simulink model "timer_load_8bit"  (R2016a)
settings: Solver=VariableStepAuto  StartTime=0.0  StopTime=1028  RelTol=1e-3
libraries: simulink_extras x9
settings Model: Creator=Cosmin  LastModifiedBy=Cosmin

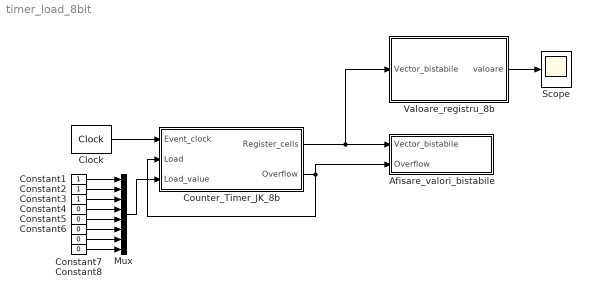
== system timer_load_8bit ==
  Afisare_valori_bistabile : Subsystem
  Clock : simulink_extras/Flip Flops/Clock  period=2
  Constant1 : Constant  OutDataTypeStr=boolean
  Constant2 : Constant  OutDataTypeStr=boolean
  Constant3 : Constant  OutDataTypeStr=boolean
  Constant{4..8} (5 alike) : Constant  Value=0  OutDataTypeStr=boolean
  Counter_Timer_JK_8b : Subsystem
  Mux : Mux  Inputs=8
  Scope : Scope
  Valoare_registru_8b : Subsystem
  wires:
  Valoare_registru_8b/1(valoare) -> Scope/1
  Counter_Timer_JK_8b/1(Register_cells) -> Afisare_valori_bistabile/1(Vector_bistabile), Valoare_registru_8b/1(Vector_bistabile)
  Clock/1 -> Counter_Timer_JK_8b/1(Event_clock)
  Counter_Timer_JK_8b/2(Overflow) -> Counter_Timer_JK_8b/2(Load), Afisare_valori_bistabile/2("Overflow ")
  Constant1/1 -> Mux/1
  Constant2/1 -> Mux/2
  Constant4/1 -> Mux/4
  Constant3/1 -> Mux/3
  Constant6/1 -> Mux/6
  Constant8/1 -> Mux/8
  Constant7/1 -> Mux/7
  Constant5/1 -> Mux/5
  Mux/1 -> Counter_Timer_JK_8b/3(Load_value)

== system timer_load_8bit/Afisare_valori_bistabile ==
  Vector_bistabile : Inport
  "Overflow " : Inport  Port=2
  Demux1 : Demux  Outputs=8
  Evolutie_bistabile_registru : Scope  NumInputPorts=9
  wires:
  Vector_bistabile/1 -> Demux1/1
  Demux1/4 -> Evolutie_bistabile_registru/4
  Demux1/2 -> Evolutie_bistabile_registru/2
  Demux1/1 -> Evolutie_bistabile_registru/1
  Demux1/3 -> Evolutie_bistabile_registru/3
  Demux1/7 -> Evolutie_bistabile_registru/7
  Demux1/5 -> Evolutie_bistabile_registru/5
  Demux1/6 -> Evolutie_bistabile_registru/6
  Demux1/8 -> Evolutie_bistabile_registru/8
  "Overflow "/1 -> Evolutie_bistabile_registru/9

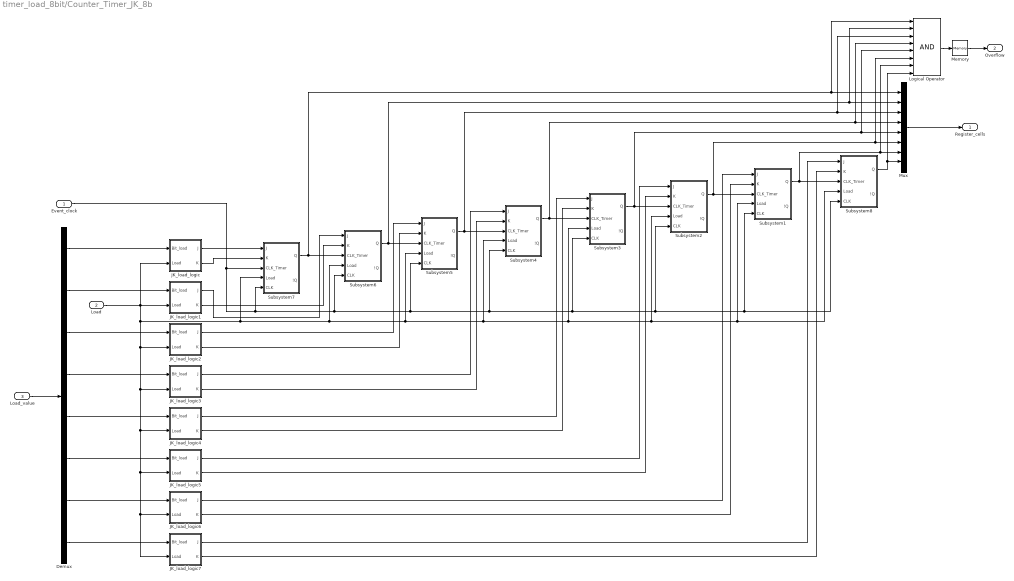
== system timer_load_8bit/Counter_Timer_JK_8b ==
  Event_clock : Inport
  Load : Inport  Port=2
  Load_value : Inport  Port=3
  Demux : Demux  Outputs=8
  JK_load_logic : Subsystem
  JK_load_logic1 : Subsystem
  JK_load_logic2 : Subsystem
  JK_load_logic3 : Subsystem
  JK_load_logic4 : Subsystem
  JK_load_logic5 : Subsystem
  JK_load_logic6 : Subsystem
  JK_load_logic7 : Subsystem
  Logical Operator : Logic  Inputs=8  AllPortsSameDT=off  OutDataTypeStr=boolean
  Memory : Memory
  Mux : Mux  Inputs=8
  Subsystem1 : Subsystem
  Subsystem2 : Subsystem
  Subsystem3 : Subsystem
  Subsystem4 : Subsystem
  Subsystem5 : Subsystem
  Subsystem6 : Subsystem
  Subsystem7 : Subsystem
  Subsystem8 : Subsystem
  Register_cells : Outport
  Overflow : Outport  Port=2
  wires:
  Mux/1 -> Register_cells/1
  Load/1 -> Subsystem7/4(Load), Subsystem6/4(Load), Subsystem5/4(Load), Subsystem4/4(Load), Subsystem3/4(Load), Subsystem2/4(Load), Subsystem8/4(Load), Subsystem1/4(Load), JK_load_logic2/2(Load), JK_load_logic3/2(Load), JK_load_logic4/2(Load), JK_load_logic5/2(Load), JK_load_logic7/2(Load), JK_load_logic6/2(Load), JK_load_logic/2(Load), JK_load_logic1/2(Load)
  Event_clock/1 -> Subsystem7/3(CLK_Timer), Subsystem7/5(CLK), Subsystem6/5(CLK), Subsystem5/5(CLK), Subsystem4/5(CLK), Subsystem3/5(CLK), Subsystem2/5(CLK), Subsystem8/5(CLK), Subsystem1/5(CLK)
  Load_value/1 -> Demux/1
  Demux/1 -> JK_load_logic/1(Bit_load)
  Demux/2 -> JK_load_logic1/1(Bit_load)
  Demux/3 -> JK_load_logic2/1(Bit_load)
  Demux/4 -> JK_load_logic3/1(Bit_load)
  Demux/5 -> JK_load_logic4/1(Bit_load)
  Demux/6 -> JK_load_logic5/1(Bit_load)
  Demux/7 -> JK_load_logic6/1(Bit_load)
  Demux/8 -> JK_load_logic7/1(Bit_load)
  JK_load_logic6/1(J) -> Subsystem1/1(J)
  JK_load_logic7/2(K) -> Subsystem8/2(K)
  JK_load_logic7/1(J) -> Subsystem8/1(J)
  Logical Operator/1 -> Memory/1
  Subsystem8/1(Q) -> Logical Operator/8, Mux/8
  Subsystem1/1(Q) -> Subsystem8/3(CLK_Timer), Logical Operator/7, Mux/7
  Subsystem2/1(Q) -> Logical Operator/6, Mux/6, Subsystem1/3(CLK_Timer)
  JK_load_logic6/2(K) -> Subsystem1/2(K)
  JK_load_logic5/1(J) -> Subsystem2/1(J)
  JK_load_logic5/2(K) -> Subsystem2/2(K)
  Subsystem3/1(Q) -> Subsystem2/3(CLK_Timer), Mux/5, Logical Operator/5
  JK_load_logic4/1(J) -> Subsystem3/1(J)
  JK_load_logic4/2(K) -> Subsystem3/2(K)
  Subsystem4/1(Q) -> Subsystem3/3(CLK_Timer), Mux/4, Logical Operator/4
  JK_load_logic3/1(J) -> Subsystem4/1(J)
  JK_load_logic3/2(K) -> Subsystem4/2(K)
  Subsystem5/1(Q) -> Subsystem4/3(CLK_Timer), Mux/3, Logical Operator/3
  JK_load_logic2/1(J) -> Subsystem5/1(J)
  JK_load_logic2/2(K) -> Subsystem5/2(K)
  Subsystem6/1(Q) -> Subsystem5/3(CLK_Timer), Logical Operator/2, Mux/2
  Subsystem7/1(Q) -> Subsystem6/3(CLK_Timer), Mux/1, Logical Operator/1
  JK_load_logic1/1(J) -> Subsystem6/1(J)
  JK_load_logic1/2(K) -> Subsystem6/2(K)
  JK_load_logic/1(J) -> Subsystem7/1(J)
  JK_load_logic/2(K) -> Subsystem7/2(K)
  Memory/1 -> Overflow/1

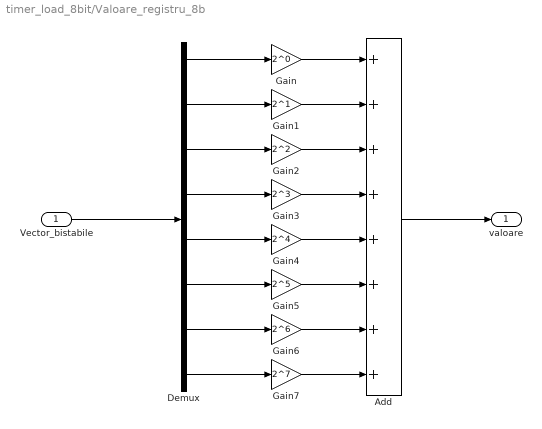
== system timer_load_8bit/Valoare_registru_8b ==
  Vector_bistabile : Inport
  Add : Sum  Inputs=++++++++
  Demux : Demux  Outputs=8
  Gain : Gain  Gain=2^0  OutDataTypeStr=uint8
  Gain1 : Gain  Gain=2^1  OutDataTypeStr=uint8
  Gain2 : Gain  Gain=2^2  OutDataTypeStr=uint8
  Gain3 : Gain  Gain=2^3  OutDataTypeStr=uint8
  Gain4 : Gain  Gain=2^4  OutDataTypeStr=uint8
  Gain5 : Gain  Gain=2^5  OutDataTypeStr=uint8
  Gain6 : Gain  Gain=2^6  OutDataTypeStr=uint8
  Gain7 : Gain  Gain=2^7  OutDataTypeStr=uint8
  valoare : Outport
  wires:
  Demux/1 -> Gain/1
  Demux/6 -> Gain5/1
  Demux/7 -> Gain6/1
  Demux/2 -> Gain1/1
  Demux/5 -> Gain4/1
  Gain5/1 -> Add/6
  Gain6/1 -> Add/7
  Gain2/1 -> Add/3
  Gain4/1 -> Add/5
  Gain3/1 -> Add/4
  Gain7/1 -> Add/8
  Gain1/1 -> Add/2
  Gain/1 -> Add/1
  Vector_bistabile/1 -> Demux/1
  Demux/3 -> Gain2/1
  Demux/4 -> Gain3/1
  Demux/8 -> Gain7/1
  Add/1 -> valoare/1

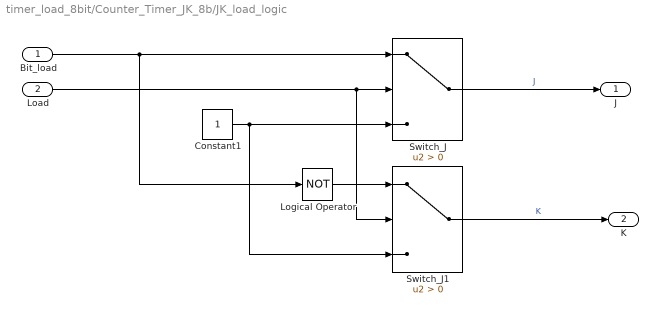
== system timer_load_8bit/Counter_Timer_JK_8b/JK_load_logic ==
  Bit_load : Inport
  Load : Inport  Port=2
  Constant1 : Constant  OutDataTypeStr=boolean
  Logical Operator : Logic  Operator=NOT  AllPortsSameDT=off  OutDataTypeStr=boolean
  Switch_J : Switch  Criteria=u2 > Threshold  OutDataTypeStr=Inherit: Inherit via back propagation
  Switch_J1 : Switch  Criteria=u2 > Threshold  OutDataTypeStr=Inherit: Inherit via back propagation
  J : Outport  OutDataTypeStr=boolean
  K : Outport  Port=2  OutDataTypeStr=boolean
  wires:
  Switch_J/1 -> J/1  "J"
  Bit_load/1 -> Logical Operator/1, Switch_J/1
  Logical Operator/1 -> Switch_J1/1
  Load/1 -> Switch_J1/2, Switch_J/2
  Constant1/1 -> Switch_J1/3, Switch_J/3
  Switch_J1/1 -> K/1  "K"

== system timer_load_8bit/Counter_Timer_JK_8b/JK_load_logic1 ==
  Bit_load : Inport
  Load : Inport  Port=2
  Constant1 : Constant  OutDataTypeStr=boolean
  Logical Operator : Logic  Operator=NOT  AllPortsSameDT=off  OutDataTypeStr=boolean
  Switch_J : Switch  Criteria=u2 > Threshold
  Switch_J1 : Switch  Criteria=u2 > Threshold
  J : Outport
  K : Outport  Port=2
  wires:
  Switch_J1/1 -> K/1  "K"
  Constant1/1 -> Switch_J/3, Switch_J1/3
  Load/1 -> Switch_J/2, Switch_J1/2
  Logical Operator/1 -> Switch_J1/1
  Bit_load/1 -> Switch_J/1, Logical Operator/1
  Switch_J/1 -> J/1  "J"

== system timer_load_8bit/Counter_Timer_JK_8b/JK_load_logic2 ==
  Bit_load : Inport
  Load : Inport  Port=2
  Constant1 : Constant  OutDataTypeStr=boolean
  Logical Operator : Logic  Operator=NOT  AllPortsSameDT=off  OutDataTypeStr=boolean
  Switch_J : Switch  Criteria=u2 > Threshold
  Switch_J1 : Switch  Criteria=u2 > Threshold
  J : Outport
  K : Outport  Port=2
  wires:
  Switch_J/1 -> J/1  "J"
  Bit_load/1 -> Logical Operator/1, Switch_J/1
  Logical Operator/1 -> Switch_J1/1
  Load/1 -> Switch_J1/2, Switch_J/2
  Constant1/1 -> Switch_J1/3, Switch_J/3
  Switch_J1/1 -> K/1  "K"

== system timer_load_8bit/Counter_Timer_JK_8b/JK_load_logic3 ==
  Bit_load : Inport
  Load : Inport  Port=2
  Constant1 : Constant  OutDataTypeStr=boolean
  Logical Operator : Logic  Operator=NOT  AllPortsSameDT=off  OutDataTypeStr=boolean
  Switch_J : Switch  Criteria=u2 > Threshold
  Switch_J1 : Switch  Criteria=u2 > Threshold
  J : Outport
  K : Outport  Port=2
  wires:
  Switch_J1/1 -> K/1  "K"
  Constant1/1 -> Switch_J/3, Switch_J1/3
  Load/1 -> Switch_J/2, Switch_J1/2
  Logical Operator/1 -> Switch_J1/1
  Bit_load/1 -> Switch_J/1, Logical Operator/1
  Switch_J/1 -> J/1  "J"

== system timer_load_8bit/Counter_Timer_JK_8b/JK_load_logic4 ==
  Bit_load : Inport
  Load : Inport  Port=2
  Constant1 : Constant  OutDataTypeStr=boolean
  Logical Operator : Logic  Operator=NOT  AllPortsSameDT=off  OutDataTypeStr=boolean
  Switch_J : Switch  Criteria=u2 > Threshold
  Switch_J1 : Switch  Criteria=u2 > Threshold
  J : Outport
  K : Outport  Port=2
  wires:
  Switch_J1/1 -> K/1  "K"
  Constant1/1 -> Switch_J/3, Switch_J1/3
  Load/1 -> Switch_J/2, Switch_J1/2
  Logical Operator/1 -> Switch_J1/1
  Bit_load/1 -> Switch_J/1, Logical Operator/1
  Switch_J/1 -> J/1  "J"

== system timer_load_8bit/Counter_Timer_JK_8b/JK_load_logic5 ==
  Bit_load : Inport
  Load : Inport  Port=2
  Constant1 : Constant  OutDataTypeStr=boolean
  Logical Operator : Logic  Operator=NOT  AllPortsSameDT=off  OutDataTypeStr=boolean
  Switch_J : Switch  Criteria=u2 > Threshold
  Switch_J1 : Switch  Criteria=u2 > Threshold
  J : Outport
  K : Outport  Port=2
  wires:
  Switch_J/1 -> J/1  "J"
  Bit_load/1 -> Logical Operator/1, Switch_J/1
  Logical Operator/1 -> Switch_J1/1
  Load/1 -> Switch_J1/2, Switch_J/2
  Constant1/1 -> Switch_J1/3, Switch_J/3
  Switch_J1/1 -> K/1  "K"

== system timer_load_8bit/Counter_Timer_JK_8b/JK_load_logic6 ==
  Bit_load : Inport
  Load : Inport  Port=2
  Constant1 : Constant  OutDataTypeStr=boolean
  Logical Operator : Logic  Operator=NOT  AllPortsSameDT=off  OutDataTypeStr=boolean
  Switch_J : Switch  Criteria=u2 > Threshold
  Switch_J1 : Switch  Criteria=u2 > Threshold
  J : Outport
  K : Outport  Port=2
  wires:
  Switch_J1/1 -> K/1  "K"
  Constant1/1 -> Switch_J/3, Switch_J1/3
  Load/1 -> Switch_J/2, Switch_J1/2
  Logical Operator/1 -> Switch_J1/1
  Bit_load/1 -> Switch_J/1, Logical Operator/1
  Switch_J/1 -> J/1  "J"

== system timer_load_8bit/Counter_Timer_JK_8b/JK_load_logic7 ==
  Bit_load : Inport
  Load : Inport  Port=2
  Constant1 : Constant  OutDataTypeStr=boolean
  Logical Operator : Logic  Operator=NOT  AllPortsSameDT=off  OutDataTypeStr=boolean
  Switch_J : Switch  Criteria=u2 > Threshold
  Switch_J1 : Switch  Criteria=u2 > Threshold
  J : Outport
  K : Outport  Port=2
  wires:
  Switch_J/1 -> J/1  "J"
  Bit_load/1 -> Logical Operator/1, Switch_J/1
  Logical Operator/1 -> Switch_J1/1
  Load/1 -> Switch_J1/2, Switch_J/2
  Constant1/1 -> Switch_J1/3, Switch_J/3
  Switch_J1/1 -> K/1  "K"

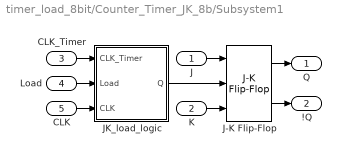
== system timer_load_8bit/Counter_Timer_JK_8b/Subsystem1 ==
  J : Inport
  K : Inport  Port=2
  CLK_Timer : Inport  Port=3
  Load : Inport  Port=4
  CLK : Inport  Port=5
  J-K Flip-Flop : simulink_extras/Flip Flops/J-K Flip-Flop  initial_condition=0
  JK_load_logic : Subsystem
  Q : Outport
  !Q : Outport  Port=2
  wires:
  J-K Flip-Flop/2 -> !Q/1
  K/1 -> J-K Flip-Flop/3
  CLK/1 -> JK_load_logic/3(CLK)
  J-K Flip-Flop/1 -> Q/1
  CLK_Timer/1 -> JK_load_logic/1(CLK_Timer)
  J/1 -> J-K Flip-Flop/1
  Load/1 -> JK_load_logic/2(Load)
  JK_load_logic/1(Q) -> J-K Flip-Flop/2

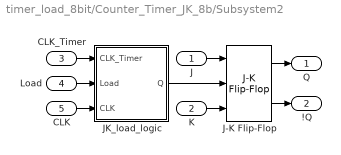
== system timer_load_8bit/Counter_Timer_JK_8b/Subsystem2 ==
  J : Inport
  K : Inport  Port=2
  CLK_Timer : Inport  Port=3
  Load : Inport  Port=4
  CLK : Inport  Port=5
  J-K Flip-Flop : simulink_extras/Flip Flops/J-K Flip-Flop  initial_condition=0
  JK_load_logic : Subsystem
  Q : Outport
  !Q : Outport  Port=2
  wires:
  JK_load_logic/1(Q) -> J-K Flip-Flop/2
  Load/1 -> JK_load_logic/2(Load)
  J/1 -> J-K Flip-Flop/1
  CLK_Timer/1 -> JK_load_logic/1(CLK_Timer)
  J-K Flip-Flop/1 -> Q/1
  CLK/1 -> JK_load_logic/3(CLK)
  K/1 -> J-K Flip-Flop/3
  J-K Flip-Flop/2 -> !Q/1

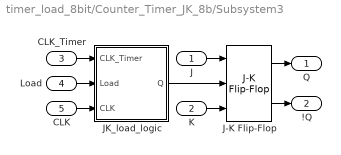
== system timer_load_8bit/Counter_Timer_JK_8b/Subsystem3 ==
  J : Inport
  K : Inport  Port=2
  CLK_Timer : Inport  Port=3
  Load : Inport  Port=4
  CLK : Inport  Port=5
  J-K Flip-Flop : simulink_extras/Flip Flops/J-K Flip-Flop  initial_condition=0
  JK_load_logic : Subsystem
  Q : Outport
  !Q : Outport  Port=2
  wires:
  J-K Flip-Flop/2 -> !Q/1
  K/1 -> J-K Flip-Flop/3
  CLK/1 -> JK_load_logic/3(CLK)
  J-K Flip-Flop/1 -> Q/1
  CLK_Timer/1 -> JK_load_logic/1(CLK_Timer)
  J/1 -> J-K Flip-Flop/1
  Load/1 -> JK_load_logic/2(Load)
  JK_load_logic/1(Q) -> J-K Flip-Flop/2

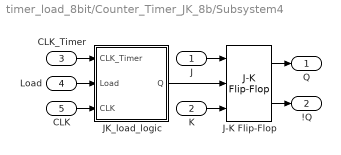
== system timer_load_8bit/Counter_Timer_JK_8b/Subsystem4 ==
  J : Inport
  K : Inport  Port=2
  CLK_Timer : Inport  Port=3
  Load : Inport  Port=4
  CLK : Inport  Port=5
  J-K Flip-Flop : simulink_extras/Flip Flops/J-K Flip-Flop  initial_condition=0
  JK_load_logic : Subsystem
  Q : Outport
  !Q : Outport  Port=2
  wires:
  JK_load_logic/1(Q) -> J-K Flip-Flop/2
  Load/1 -> JK_load_logic/2(Load)
  J/1 -> J-K Flip-Flop/1
  CLK_Timer/1 -> JK_load_logic/1(CLK_Timer)
  J-K Flip-Flop/1 -> Q/1
  CLK/1 -> JK_load_logic/3(CLK)
  K/1 -> J-K Flip-Flop/3
  J-K Flip-Flop/2 -> !Q/1

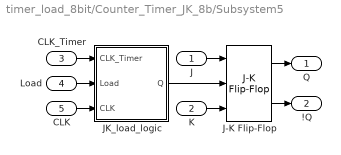
== system timer_load_8bit/Counter_Timer_JK_8b/Subsystem5 ==
  J : Inport
  K : Inport  Port=2
  CLK_Timer : Inport  Port=3
  Load : Inport  Port=4
  CLK : Inport  Port=5
  J-K Flip-Flop : simulink_extras/Flip Flops/J-K Flip-Flop  initial_condition=0
  JK_load_logic : Subsystem
  Q : Outport
  !Q : Outport  Port=2
  wires:
  J-K Flip-Flop/2 -> !Q/1
  K/1 -> J-K Flip-Flop/3
  CLK/1 -> JK_load_logic/3(CLK)
  J-K Flip-Flop/1 -> Q/1
  CLK_Timer/1 -> JK_load_logic/1(CLK_Timer)
  J/1 -> J-K Flip-Flop/1
  Load/1 -> JK_load_logic/2(Load)
  JK_load_logic/1(Q) -> J-K Flip-Flop/2

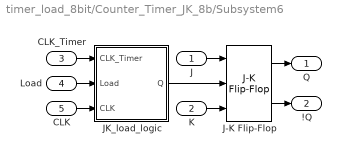
== system timer_load_8bit/Counter_Timer_JK_8b/Subsystem6 ==
  J : Inport
  K : Inport  Port=2
  CLK_Timer : Inport  Port=3
  Load : Inport  Port=4
  CLK : Inport  Port=5
  J-K Flip-Flop : simulink_extras/Flip Flops/J-K Flip-Flop  initial_condition=0
  JK_load_logic : Subsystem
  Q : Outport
  !Q : Outport  Port=2
  wires:
  JK_load_logic/1(Q) -> J-K Flip-Flop/2
  Load/1 -> JK_load_logic/2(Load)
  J/1 -> J-K Flip-Flop/1
  CLK_Timer/1 -> JK_load_logic/1(CLK_Timer)
  J-K Flip-Flop/1 -> Q/1
  CLK/1 -> JK_load_logic/3(CLK)
  K/1 -> J-K Flip-Flop/3
  J-K Flip-Flop/2 -> !Q/1

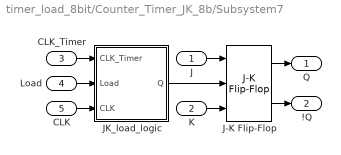
== system timer_load_8bit/Counter_Timer_JK_8b/Subsystem7 ==
  J : Inport
  K : Inport  Port=2
  CLK_Timer : Inport  Port=3
  Load : Inport  Port=4
  CLK : Inport  Port=5
  J-K Flip-Flop : simulink_extras/Flip Flops/J-K Flip-Flop  initial_condition=0
  JK_load_logic : Subsystem
  Q : Outport
  !Q : Outport  Port=2
  wires:
  J-K Flip-Flop/2 -> !Q/1
  K/1 -> J-K Flip-Flop/3
  CLK/1 -> JK_load_logic/3(CLK)
  J-K Flip-Flop/1 -> Q/1
  CLK_Timer/1 -> JK_load_logic/1(CLK_Timer)
  J/1 -> J-K Flip-Flop/1
  Load/1 -> JK_load_logic/2(Load)
  JK_load_logic/1(Q) -> J-K Flip-Flop/2

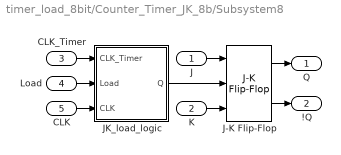
== system timer_load_8bit/Counter_Timer_JK_8b/Subsystem8 ==
  J : Inport
  K : Inport  Port=2
  CLK_Timer : Inport  Port=3
  Load : Inport  Port=4
  CLK : Inport  Port=5
  J-K Flip-Flop : simulink_extras/Flip Flops/J-K Flip-Flop  initial_condition=0
  JK_load_logic : Subsystem
  Q : Outport
  !Q : Outport  Port=2
  wires:
  JK_load_logic/1(Q) -> J-K Flip-Flop/2
  Load/1 -> JK_load_logic/2(Load)
  J/1 -> J-K Flip-Flop/1
  CLK_Timer/1 -> JK_load_logic/1(CLK_Timer)
  J-K Flip-Flop/1 -> Q/1
  CLK/1 -> JK_load_logic/3(CLK)
  K/1 -> J-K Flip-Flop/3
  J-K Flip-Flop/2 -> !Q/1

== system timer_load_8bit/Counter_Timer_JK_8b/Subsystem1/JK_load_logic ==
  CLK_Timer : Inport
  Load : Inport  Port=2
  CLK : Inport  Port=3
  Switch_J : Switch  Criteria=u2 > Threshold  Threshold=0.5  OutDataTypeStr=uint8
  Q : Outport
  wires:
  Load/1 -> Switch_J/2
  Switch_J/1 -> Q/1  "J"
  CLK/1 -> Switch_J/1
  CLK_Timer/1 -> Switch_J/3

== system timer_load_8bit/Counter_Timer_JK_8b/Subsystem2/JK_load_logic ==
  CLK_Timer : Inport
  Load : Inport  Port=2
  CLK : Inport  Port=3
  Switch_J : Switch  Criteria=u2 > Threshold  Threshold=0.5  OutDataTypeStr=uint8
  Q : Outport
  wires:
  CLK_Timer/1 -> Switch_J/3
  CLK/1 -> Switch_J/1
  Switch_J/1 -> Q/1  "J"
  Load/1 -> Switch_J/2

== system timer_load_8bit/Counter_Timer_JK_8b/Subsystem3/JK_load_logic ==
  CLK_Timer : Inport
  Load : Inport  Port=2
  CLK : Inport  Port=3
  Switch_J : Switch  Criteria=u2 > Threshold  Threshold=0.5  OutDataTypeStr=uint8
  Q : Outport
  wires:
  Load/1 -> Switch_J/2
  Switch_J/1 -> Q/1  "J"
  CLK/1 -> Switch_J/1
  CLK_Timer/1 -> Switch_J/3

== system timer_load_8bit/Counter_Timer_JK_8b/Subsystem4/JK_load_logic ==
  CLK_Timer : Inport
  Load : Inport  Port=2
  CLK : Inport  Port=3
  Switch_J : Switch  Criteria=u2 > Threshold  Threshold=0.5  OutDataTypeStr=uint8
  Q : Outport
  wires:
  CLK_Timer/1 -> Switch_J/3
  CLK/1 -> Switch_J/1
  Switch_J/1 -> Q/1  "J"
  Load/1 -> Switch_J/2

== system timer_load_8bit/Counter_Timer_JK_8b/Subsystem5/JK_load_logic ==
  CLK_Timer : Inport
  Load : Inport  Port=2
  CLK : Inport  Port=3
  Switch_J : Switch  Criteria=u2 > Threshold  Threshold=0.5  OutDataTypeStr=uint8
  Q : Outport
  wires:
  Load/1 -> Switch_J/2
  Switch_J/1 -> Q/1  "J"
  CLK/1 -> Switch_J/1
  CLK_Timer/1 -> Switch_J/3

== system timer_load_8bit/Counter_Timer_JK_8b/Subsystem6/JK_load_logic ==
  CLK_Timer : Inport
  Load : Inport  Port=2
  CLK : Inport  Port=3
  Switch_J : Switch  Criteria=u2 > Threshold  Threshold=0.5  OutDataTypeStr=uint8
  Q : Outport
  wires:
  CLK_Timer/1 -> Switch_J/3
  CLK/1 -> Switch_J/1
  Switch_J/1 -> Q/1  "J"
  Load/1 -> Switch_J/2

== system timer_load_8bit/Counter_Timer_JK_8b/Subsystem7/JK_load_logic ==
  CLK_Timer : Inport
  Load : Inport  Port=2
  CLK : Inport  Port=3
  Switch_J : Switch  Criteria=u2 > Threshold  Threshold=0.5  OutDataTypeStr=uint8
  Q : Outport
  wires:
  Load/1 -> Switch_J/2
  Switch_J/1 -> Q/1  "J"
  CLK/1 -> Switch_J/1
  CLK_Timer/1 -> Switch_J/3

== system timer_load_8bit/Counter_Timer_JK_8b/Subsystem8/JK_load_logic ==
  CLK_Timer : Inport
  Load : Inport  Port=2
  CLK : Inport  Port=3
  Switch_J : Switch  Criteria=u2 > Threshold  Threshold=0.5  OutDataTypeStr=uint8
  Q : Outport
  wires:
  CLK_Timer/1 -> Switch_J/3
  CLK/1 -> Switch_J/1
  Switch_J/1 -> Q/1  "J"
  Load/1 -> Switch_J/2
